simulink model "motor2"  (Simulink 7.3)
settings: Solver=ode45  StartTime=0.0  StopTime=10  RelTol=1e-3
values from neighbouring files (symbols this model uses):
  Beq = 0.0015    [Sve_ikad.m]    (also in matlab.mat)
  Eff_G = 0.9    [Sve_ikad.m]    (also in matlab.mat)
  Eff_M = 0.69    [Sve_ikad.m]    (also in matlab.mat)
  Jeq = 9.785e-5    (= 9.785e-05)    [Sve_ikad.m]    (also in matlab.mat)
  Ke = 0.0076776    [Sve_ikad.m]    (also in matlab.mat)
  Kg = 14    [Sve_ikad.m]    (also in matlab.mat)
  Km = 0.007683    [Sve_ikad.m]    (also in matlab.mat)
  Ra = 2.6    [Sve_ikad.m]    (also in matlab.mat)
settings Model: Creator=Labos  LastModifiedBy=Labos

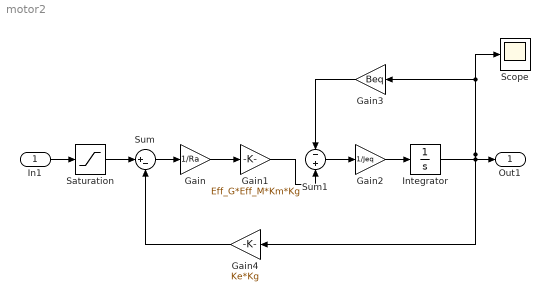
== system motor2 ==
  In1 : Inport  OutDataType=fixdt(1, 16)  OutScaling=2^0
  Gain : Gain  Gain=1/Ra  ParameterDataType=fixdt(1, 16)  ParameterScaling=2^0  OutDataType=fixdt(1, 16)  OutScaling=2^0
  Gain1 : Gain  Gain=Eff_G*Eff_M*Km*Kg  ParameterDataType=fixdt(1, 16)  ParameterScaling=2^0  OutDataType=fixdt(1, 16)  OutScaling=2^0
  Gain2 : Gain  Gain=1/Jeq  ParameterDataType=fixdt(1, 16)  ParameterScaling=2^0  OutDataType=fixdt(1, 16)  OutScaling=2^0
  Gain3 : Gain  Gain=Beq  ParameterDataType=fixdt(1, 16)  ParameterScaling=2^0  OutDataType=fixdt(1, 16)  OutScaling=2^0
  Gain4 : Gain  Gain=Ke*Kg  ParameterDataType=fixdt(1, 16)  ParameterScaling=2^0  OutDataType=fixdt(1, 16)  OutScaling=2^0
  Integrator : Integrator
  Saturation : Saturate  UpperLimit=6  LowerLimit=-6  OutDataType=fixdt(1, 16)  OutScaling=2^0
  Scope : Scope
  Sum : Sum  Inputs=|+-  OutDataType=fixdt(1, 16)  OutScaling=2^0
  Sum1 : Sum  Inputs=-+  OutDataType=fixdt(1, 16)  OutScaling=2^0
  Out1 : Outport  OutDataType=fixdt(1, 16)  OutScaling=2^0
  wires:
  In1/1 -> Saturation/1
  Saturation/1 -> Sum/1
  Sum/1 -> Gain/1
  Gain/1 -> Gain1/1
  Sum1/1 -> Gain2/1
  Gain1/1 -> Sum1/2
  Gain3/1 -> Sum1/1
  Gain4/1 -> Sum/2
  Gain2/1 -> Integrator/1
  Integrator/1 -> Out1/1, Gain4/1, Gain3/1, Scope/1
